simulink model "simplethreephasemodel_expanded_balanced"  (R2017b)
settings: Solver=VariableStepAuto  StartTime=0.0  StopTime=0.1  RelTol=1e-3
libraries: pe_lib x7, fl_lib x4, nesl_utility x3
settings Model: Creator=hansmariushagen  LastModifiedBy=hansmariushagen

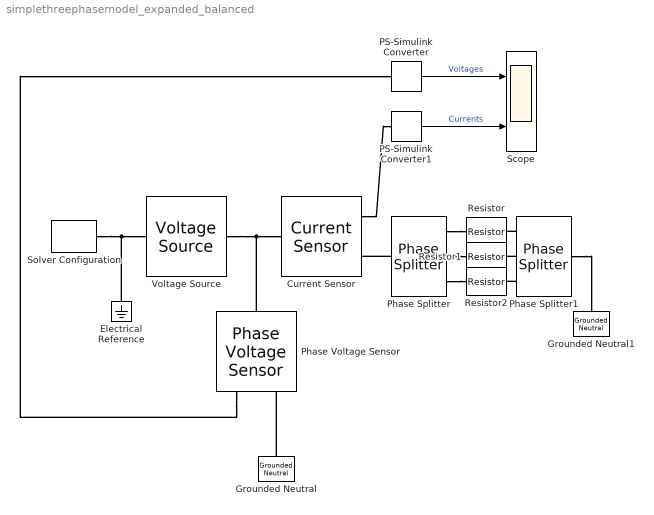
== system simplethreephasemodel_expanded_balanced ==
  Current Sensor : pe_lib/Sensors/Current Sensor
      settings: SourceProductName=Simscape Power Systems  SourceProductBaseCode=PS
  Electrical Reference : fl_lib/Electrical/Electrical Elements/Electrical Reference
  Grounded Neutral : pe_lib/Connections/Grounded Neutral
      settings: SourceProductName=Simscape Power Systems  SourceProductBaseCode=PS
  Grounded Neutral1 : pe_lib/Connections/Grounded Neutral
      settings: SourceProductName=Simscape Power Systems  SourceProductBaseCode=PS
  PS-Simulink Converter : nesl_utility/PS-Simulink Converter  PhysicalDomain=network_engine_domain  SubClassName=ps_output  LeftPortType=input  RightPortType=output  PseudoPeriodic=off  Frequencies=[]  Unit=V  AffineConversion=off
  PS-Simulink Converter1 : nesl_utility/PS-Simulink Converter  PhysicalDomain=network_engine_domain  SubClassName=ps_output  LeftPortType=input  RightPortType=output  PseudoPeriodic=off  Frequencies=[]  Unit=A  AffineConversion=off
  Phase Splitter : pe_lib/Connections/Phase Splitter
      settings: SourceProductName=Simscape Power Systems  SourceProductBaseCode=PS
  Phase Splitter1 : pe_lib/Connections/Phase Splitter
      settings: SourceProductName=Simscape Power Systems  SourceProductBaseCode=PS
  Phase Voltage Sensor : pe_lib/Sensors/Phase Voltage Sensor
      settings: SourceProductName=Simscape Power Systems  SourceProductBaseCode=PS
  Resistor : fl_lib/Electrical/Electrical Elements/Resistor  R=1 Ohm  i_specify=off  i_priority=None  i=0 A  i_nominal_specify=off  i_nominal_unit=A  i_nominal_value=1  v_specify=off  v_priority=None  v=0 V  v_nominal_specify=off  v_nominal_unit=V  v_nominal_value=1
  Resistor1 : fl_lib/Electrical/Electrical Elements/Resistor  R=1 Ohm  i_specify=off  i_priority=None  i=0 A  i_nominal_specify=off  i_nominal_unit=A  i_nominal_value=1  v_specify=off  v_priority=None  v=0 V  v_nominal_specify=off  v_nominal_unit=V  v_nominal_value=1
  Resistor2 : fl_lib/Electrical/Electrical Elements/Resistor  R=1 Ohm  i_specify=off  i_priority=None  i=0 A  i_nominal_specify=off  i_nominal_unit=A  i_nominal_value=1  v_specify=off  v_priority=None  v=0 V  v_nominal_specify=off  v_nominal_unit=V  v_nominal_value=1
  Scope : Scope  NumInputPorts=2
  Solver Configuration : nesl_utility/Solver Configuration  PhysicalDomain=network_engine_domain  SubClassName=solver  LeftPortType=input  RightPortType=generic  Accelerate=off  Tones=[]  Harmonics=[]  SimulateNoise=off  Profile=off  UseLocalSampling=off  EnableSwitchedLinearOptims=on  FrequencyDomain=off  UseCCode=off  RelTol=0.001  AbsTol=1e-06  MinStep=1e-09  ToWorkspace=off  RevertToSquareIcSolve=off  NumHomotopyIterations=100  PhasorMode=off  PhasorModeNumHarmonics=1  DoDC=off  ResidualTolerance=1e-09  UseLocalSolver=on  LocalSolverChoice=NE_BACKWARD_EULER_ADVANCER  LocalSolverSampleTime=0.00001  DoFixedCost=on  MaxNonlinIter=3  MaxModeIter=2  LinearAlgebra=Sparse  DelaysMemoryBudget=1024  AutomaticFiltering=on  FilteringTimeConstant=0.001
  Voltage Source : pe_lib/Sources/Voltage Source  vline_rms=sqrt(3) * 100 / sqrt(2) V  shift=0 deg  freq=60 Hz  impedance_option=1  SShortCircuit=1e6 V*A  XR=15  R=0.01 Ohm  L=3.97e-4 H  G_parasitic=0 1/Ohm  harmonic_option=0  harmonic_orders=[5, 7, 11, 13]  harmonic_ratios=[.1, .1, .1, .1]  I_specify=off  I_priority=None  I=[ 0 0 0 ] A  I_nominal_specify=off  I_nominal_unit=A  I_nominal_value=1
      settings: SourceProductName=Simscape Power Systems  SourceProductBaseCode=PS
  wires:
  PS-Simulink Converter1/1 -> Scope/2  "Currents"
  PS-Simulink Converter/1 -> Scope/1  "Voltages"
  connections:
  Current Sensor/RConn1 -- PS-Simulink Converter1/LConn1
  Phase Splitter/LConn1 -- Current Sensor/RConn2
  Phase Splitter1/LConn1 -- Grounded Neutral1/LConn1
  Voltage Source/RConn1 -- Phase Voltage Sensor/LConn1 -- Current Sensor/LConn1
  Solver Configuration/RConn1 -- Electrical Reference/LConn1 -- Voltage Source/LConn1
  Phase Voltage Sensor/RConn1 -- PS-Simulink Converter/LConn1
  Grounded Neutral/LConn1 -- Phase Voltage Sensor/RConn2
  Phase Splitter1/RConn1 -- Resistor/RConn1
  Phase Splitter1/RConn2 -- Resistor1/RConn1
  Phase Splitter1/RConn3 -- Resistor2/RConn1
  Phase Splitter/RConn1 -- Resistor/LConn1
  Phase Splitter/RConn2 -- Resistor1/LConn1
  Phase Splitter/RConn3 -- Resistor2/LConn1
